simulink model "PE_weightstationary"  (R2022a)
settings: Solver=VariableStepAuto  StartTime=0.0  StopTime=20  RelTol=1e-3
values from neighbouring files (symbols this model uses):
  eta = 0.001    [array_2x2_input.m]
  num_layer = 4    [array_2x2_input.m]
undefined symbols (not defined in the file or in its folder): xc7k70tfbv676
libraries: hdlBasic x77, vmcUtilities x1
(part 1 of 2)
settings Model: Creator=gaozh  LastModifiedBy=gaozh

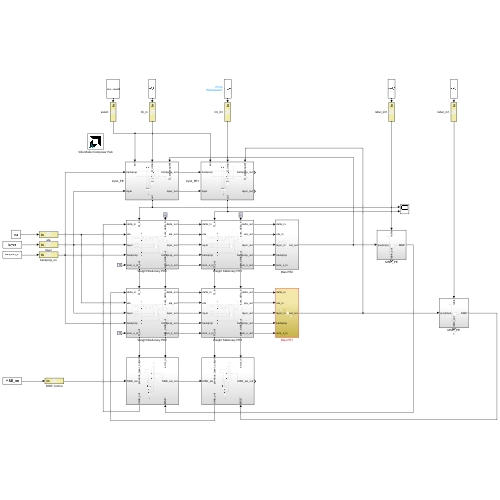
[thumbnail: Simulink's stored preview of the top-level diagram]
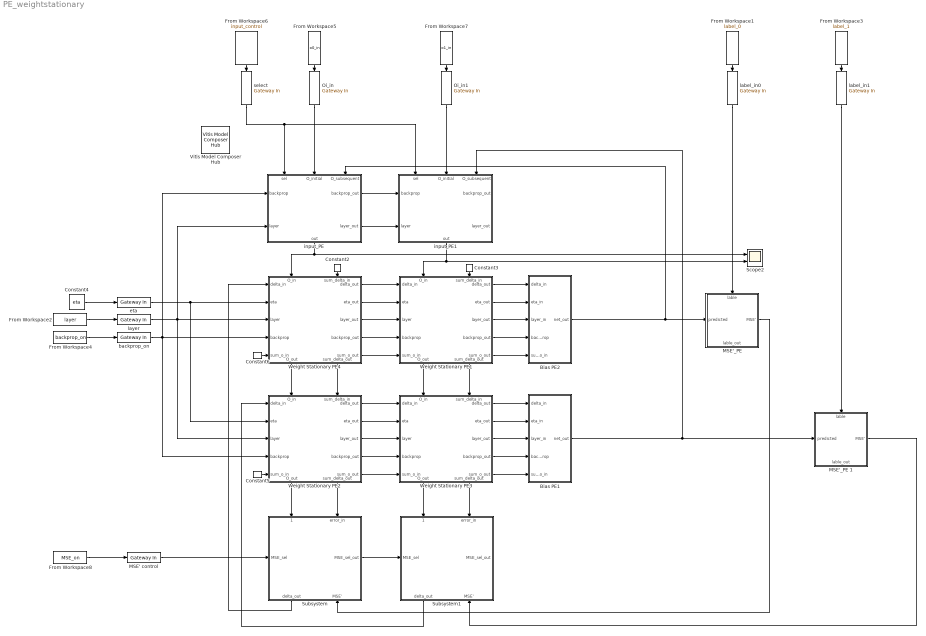
== system PE_weightstationary ==
  Bias PE1 : Subsystem
  Bias PE2 : Subsystem
  Constant{2..3,5..6} (4 alike) : hdlBasic/Constant  const=0  gui_display_data_type=Fixed-point  arith_type=Signed (2's comp)  n_bits=num_bits  bin_pt=frac_bits  preci_type=Single  exp_width=8  frac_width=24  explicit_period=off  period=1  XmcBlockStatus=1  maskContainerNames=tabcontainer1  block_type=constant  block_config=sysgen:Constant_config
  Constant4 : Constant  Value=eta
  From Workspace1 : FromWorkspace  VariableName=label_0
  From Workspace2 : FromWorkspace  VariableName=layer
  From Workspace3 : FromWorkspace  VariableName=label_1
  From Workspace4 : FromWorkspace  VariableName=backprop_on
  From Workspace5 : FromWorkspace  VariableName=o0_in
  From Workspace6 : FromWorkspace  VariableName=input_control
  From Workspace7 : FromWorkspace  VariableName=o1_in
  From Workspace8 : FromWorkspace  VariableName=MSE_on
  MSE' control : hdlBasic/Gateway In  gui_display_data_type=Boolean  arith_type=Boolean  n_bits=num_bits  bin_pt=0  preci_type=Single  exp_width=8  frac_width=24  rows=1  columns=1  quantization="Round  (unbiased: +/- Inf)"  overflow=Saturate  period=1  UseAsADC=off  ADCChannel='1'  interface=None  automatic_assignment=on  address_offset=hex2dec('00')  intf_name=''  intf_description=''  default_value=0  timing_constraint=None  locs_specified=off  LOCs={}  io_standard={}  inherit_from_input=off  hdl_port=on  XmcBlockStatus=1  maskContainerNames=group4  block_type=gatewayin  block_config=sysgen:gateway_in_config  block_width_w=590  block_height_w=620  block_width=640  block_height=850
  "MSE'_PE " : Subsystem
      settings: PortSchema="{\"entries\":[{\"content\":{\"sides\":[{\"content\":{\"connectorIds\":[\"In1\"]},\"type\":\"ConnectorPlacement.EquallySpacedRectSide\",\"uuid\":\"709b04f5-809b-41cc-9440-aba08c0e6347\"},{\"content\":{\"connectorIds\":[\"Out1\"],\"side\":\"RIGHT\"},\"type\":\"ConnectorPlacement.EquallySpacedRectSide\",\"uuid\":\"2a9bc808-cd74-4923-8833-c733d5b55101\"},{\"content\":{\"connectorIds\":[\"In2\"],\"side\":\"TOP\"},\"type\":\"ConnectorPlacement.EquallySpacedRectSide\",\"uuid\":\"1b9115af-72f6-4ff5-884d-2691fdb3b6f3\"},{\"content\":{\"connectorIds\":[\"Out2\"],\"side\":\"BOTTOM\"},\"type\":\"ConnectorPlacement.EquallySpacedRectSide\",\"uuid\":\"91ceb1b5-75ad-4997-b7e4-e67318ba19d7\"}]},\"type\":\"ConnectorPlacement.EquallySpacedConnector\",\"uuid\":\"1849f986-7f00-43c7-976b-1eef01c166bf\"}],\"packageUris\":[\"http://schema.mathworks.com/mf0/Connector/R2020b\"],\"version\":\"1.0\"}"
  MSE'_PE 1 : Subsystem
      settings: PortSchema="{\"entries\":[{\"content\":{\"sides\":[{\"content\":{\"connectorIds\":[\"In1\"]},\"type\":\"ConnectorPlacement.EquallySpacedRectSide\",\"uuid\":\"709b04f5-809b-41cc-9440-aba08c0e6347\"},{\"content\":{\"connectorIds\":[\"Out1\"],\"side\":\"RIGHT\"},\"type\":\"ConnectorPlacement.EquallySpacedRectSide\",\"uuid\":\"2a9bc808-cd74-4923-8833-c733d5b55101\"},{\"content\":{\"connectorIds\":[\"In2\"],\"side\":\"TOP\"},\"type\":\"ConnectorPlacement.EquallySpacedRectSide\",\"uuid\":\"1b9115af-72f6-4ff5-884d-2691fdb3b6f3\"},{\"content\":{\"connectorIds\":[\"Out2\"],\"side\":\"BOTTOM\"},\"type\":\"ConnectorPlacement.EquallySpacedRectSide\",\"uuid\":\"91ceb1b5-75ad-4997-b7e4-e67318ba19d7\"}]},\"type\":\"ConnectorPlacement.EquallySpacedConnector\",\"uuid\":\"1849f986-7f00-43c7-976b-1eef01c166bf\"}],\"packageUris\":[\"http://schema.mathworks.com/mf0/Connector/R2020b\"],\"version\":\"1.0\"}"
  Oi_in : hdlBasic/Gateway In  gui_display_data_type=Fixed-point  arith_type=Signed (2's comp)  n_bits=num_bits  bin_pt=frac_bits  preci_type=Single  exp_width=8  frac_width=24  rows=1  columns=1  quantization="Round  (unbiased: +/- Inf)"  overflow=Saturate  period=1  UseAsADC=off  ADCChannel='1'  interface=None  automatic_assignment=on  address_offset=hex2dec('00')  intf_name=''  intf_description=''  default_value=0  timing_constraint=None  locs_specified=off  LOCs={}  io_standard={}  inherit_from_input=off  hdl_port=on  XmcBlockStatus=1  maskContainerNames=group4  block_type=gatewayin  block_config=sysgen:gateway_in_config  block_width_w=590  block_height_w=620  block_width=640  block_height=850
  Oi_in1 : hdlBasic/Gateway In  gui_display_data_type=Fixed-point  arith_type=Signed (2's comp)  n_bits=num_bits  bin_pt=frac_bits  preci_type=Single  exp_width=8  frac_width=24  rows=1  columns=1  quantization="Round  (unbiased: +/- Inf)"  overflow=Saturate  period=1  UseAsADC=off  ADCChannel='1'  interface=None  automatic_assignment=on  address_offset=hex2dec('00')  intf_name=''  intf_description=''  default_value=0  timing_constraint=None  locs_specified=off  LOCs={}  io_standard={}  inherit_from_input=off  hdl_port=on  XmcBlockStatus=1  maskContainerNames=group4  block_type=gatewayin  block_config=sysgen:gateway_in_config  block_width_w=590  block_height_w=620  block_width=640  block_height=850
  Scope2 : Scope  NumInputPorts=2
  Subsystem : Subsystem
      settings: PortSchema="{\"entries\":[{\"content\":{\"sides\":[{\"content\":{\"connectorIds\":[\"In1\",\"In2\"]},\"type\":\"ConnectorPlacement.EquallySpacedRectSide\",\"uuid\":\"dbd75916-d643-4f7d-9fb6-d710889911bc\"},{\"content\":{\"connectorIds\":[\"Out1\",\"In4\"],\"side\":\"RIGHT\"},\"type\":\"ConnectorPlacement.EquallySpacedRectSide\",\"uuid\":\"bd082d37-a6ba-4642-a234-a4ee2405f373\"},{\"content\":{\"connectorIds\":[\"In3\"],\"side\":\"TOP\"},\"type\":\"ConnectorPlacement.EquallySpacedRectSide\",\"uuid\":\"2acf0bf3-92c2-4168-859e-2b2ecd63c261\"},{\"content\":{\"connectorIds\":[\"Out2\"],\"side\":\"BOTTOM\"},\"type\":\"ConnectorPlacement.EquallySpacedRectSide\",\"uuid\":\"570ce3db-e00a-4edd-9e75-c3405427573c\"}]},\"type\":\"ConnectorPlacement.EquallySpacedConnector\",\"uuid\":\"e2ba7bdc-2926-4fef-94e6-45d12da95ba7\"}],\"packageUris\":[\"http://schema.mathworks.com/mf0/Connector/R2020b\"],\"version\":\"1.0\"}"
  Subsystem1 : Subsystem
      settings: PortSchema="{\"entries\":[{\"content\":{\"sides\":[{\"content\":{\"connectorIds\":[\"In1\",\"In2\"]},\"type\":\"ConnectorPlacement.EquallySpacedRectSide\",\"uuid\":\"dbd75916-d643-4f7d-9fb6-d710889911bc\"},{\"content\":{\"connectorIds\":[\"Out1\",\"In4\"],\"side\":\"RIGHT\"},\"type\":\"ConnectorPlacement.EquallySpacedRectSide\",\"uuid\":\"bd082d37-a6ba-4642-a234-a4ee2405f373\"},{\"content\":{\"connectorIds\":[\"In3\"],\"side\":\"TOP\"},\"type\":\"ConnectorPlacement.EquallySpacedRectSide\",\"uuid\":\"2acf0bf3-92c2-4168-859e-2b2ecd63c261\"},{\"content\":{\"connectorIds\":[\"Out2\"],\"side\":\"BOTTOM\"},\"type\":\"ConnectorPlacement.EquallySpacedRectSide\",\"uuid\":\"570ce3db-e00a-4edd-9e75-c3405427573c\"}]},\"type\":\"ConnectorPlacement.EquallySpacedConnector\",\"uuid\":\"e2ba7bdc-2926-4fef-94e6-45d12da95ba7\"}],\"packageUris\":[\"http://schema.mathworks.com/mf0/Connector/R2020b\"],\"version\":\"1.0\"}"
  Vitis Model Composer Hub : vmcUtilities/Vitis Model Composer Hub  Tag=genX  CodeGeneration=off  TargetDirectory=./code  ExportType=AI Engines  IpVendor=xilinx.com  IpLibrary=hls  IpVersion=1.0  IpHWLanguage=Verilog  AieCompilerOptions={}  AieSimulatorOptions={}  CreateTestbench=off  TestbenchStackSize=10  RunAieSim=off  AieSimTimeout=50000  RunAieSimProfiling=off  LaunchVitisAnalyzer=off  PlotOutput=off  RunX86Sim=off  X86SimTimeout=10  GenHwImage=off  PlatformType=Not Specified  HwSystemType=Baremetal  HwValidationTarget=hw  ProjDevice=xc7k70tfbv676-1  ProjDevicePart=xc7k70tfbv676-1  SamplePeriod=-1  ClockFrequency=200  DataPathParallelism=1  xilinxfamily=kintex7  part=xc7k70t  speed=-1  package=fbv676  directory=./netlist  testbench=off  incr_netlist=off  synthesis_tool=Vivado  clock_wrapper=Clock Enables  dbl_ovrd=According to Block Masks  dcm_input_clock_period=10  sysclk_period=10  simulink_period=1  eval_field=0  IPInfoJsonString="{\"HDLSubsystem\":{\"SubsystemName\":\"PE_weightstationary\",\"IPName\":\"weight_pe\",\"IPLibrary\":\"VMC\",\"IPVendor\":\"User Company\",\"IPVersion\":\"1.0\"}}"  LogFileName=''  NThreads=4
  Weight Stationary PE1 : Subsystem
      settings: PortSchema="{\"entries\":[{\"content\":{\"sides\":[{\"content\":{\"connectorIds\":[\"In1\",\"In2\",\"In3\",\"In4\",\"In5\"]},\"type\":\"ConnectorPlacement.EquallySpacedRectSide\",\"uuid\":\"632a3ded-5b94-406e-b0d8-119737680536\"},{\"content\":{\"connectorIds\":[\"Out1\",\"Out2\",\"Out3\",\"Out4\",\"Out5\"],\"side\":\"RIGHT\"},\"type\":\"ConnectorPlacement.EquallySpacedRectSide\",\"uuid\":\"c449027c-81bc-4843-8994-fcad26195520\"},{\"content\":{\"connectorIds\":[\"In6\",\"In7\"],\"side\":\"TOP\"},\"type\":\"ConnectorPlacement.EquallySpacedRectSide\",\"uuid\":\"ce3d970d-7335-434e-bfbf-286e0c492397\"},{\"content\":{\"connectorIds\":[\"Out6\",\"Out7\"],\"side\":\"BOTTOM\"},\"type\":\"ConnectorPlacement.EquallySpacedRectSide\",\"uuid\":\"bc179919-f31d-4e0a-abc3-bb5ef913c3c8\"}]},\"type\":\"ConnectorPlacement.EquallySpacedConnector\",\"uuid\":\"cad1cfc6-1bed-4a03-a2df-30ebe0a8ed6f\"}],\"packageUris\":[\"http://schema.mathworks.com/mf0/Connector/R2020b\"],\"version\":\"1.0\"}"
  Weight Stationary PE2 : Subsystem
      settings: PortSchema="{\"entries\":[{\"content\":{\"sides\":[{\"content\":{\"connectorIds\":[\"In1\",\"In2\",\"In3\",\"In4\",\"In5\"]},\"type\":\"ConnectorPlacement.EquallySpacedRectSide\",\"uuid\":\"632a3ded-5b94-406e-b0d8-119737680536\"},{\"content\":{\"connectorIds\":[\"Out1\",\"Out2\",\"Out3\",\"Out4\",\"Out5\"],\"side\":\"RIGHT\"},\"type\":\"ConnectorPlacement.EquallySpacedRectSide\",\"uuid\":\"c449027c-81bc-4843-8994-fcad26195520\"},{\"content\":{\"connectorIds\":[\"In6\",\"In7\"],\"side\":\"TOP\"},\"type\":\"ConnectorPlacement.EquallySpacedRectSide\",\"uuid\":\"ce3d970d-7335-434e-bfbf-286e0c492397\"},{\"content\":{\"connectorIds\":[\"Out6\",\"Out7\"],\"side\":\"BOTTOM\"},\"type\":\"ConnectorPlacement.EquallySpacedRectSide\",\"uuid\":\"bc179919-f31d-4e0a-abc3-bb5ef913c3c8\"}]},\"type\":\"ConnectorPlacement.EquallySpacedConnector\",\"uuid\":\"cad1cfc6-1bed-4a03-a2df-30ebe0a8ed6f\"}],\"packageUris\":[\"http://schema.mathworks.com/mf0/Connector/R2020b\"],\"version\":\"1.0\"}"
  Weight Stationary PE3 : Subsystem
      settings: PortSchema="{\"entries\":[{\"content\":{\"sides\":[{\"content\":{\"connectorIds\":[\"In1\",\"In2\",\"In3\",\"In4\",\"In5\"]},\"type\":\"ConnectorPlacement.EquallySpacedRectSide\",\"uuid\":\"632a3ded-5b94-406e-b0d8-119737680536\"},{\"content\":{\"connectorIds\":[\"Out1\",\"Out2\",\"Out3\",\"Out4\",\"Out5\"],\"side\":\"RIGHT\"},\"type\":\"ConnectorPlacement.EquallySpacedRectSide\",\"uuid\":\"c449027c-81bc-4843-8994-fcad26195520\"},{\"content\":{\"connectorIds\":[\"In6\",\"In7\"],\"side\":\"TOP\"},\"type\":\"ConnectorPlacement.EquallySpacedRectSide\",\"uuid\":\"ce3d970d-7335-434e-bfbf-286e0c492397\"},{\"content\":{\"connectorIds\":[\"Out6\",\"Out7\"],\"side\":\"BOTTOM\"},\"type\":\"ConnectorPlacement.EquallySpacedRectSide\",\"uuid\":\"bc179919-f31d-4e0a-abc3-bb5ef913c3c8\"}]},\"type\":\"ConnectorPlacement.EquallySpacedConnector\",\"uuid\":\"cad1cfc6-1bed-4a03-a2df-30ebe0a8ed6f\"}],\"packageUris\":[\"http://schema.mathworks.com/mf0/Connector/R2020b\"],\"version\":\"1.0\"}"
  Weight Stationary PE4 : Subsystem
      settings: PortSchema="{\"entries\":[{\"content\":{\"sides\":[{\"content\":{\"connectorIds\":[\"In1\",\"In2\",\"In3\",\"In4\",\"In5\"]},\"type\":\"ConnectorPlacement.EquallySpacedRectSide\",\"uuid\":\"632a3ded-5b94-406e-b0d8-119737680536\"},{\"content\":{\"connectorIds\":[\"Out1\",\"Out2\",\"Out3\",\"Out4\",\"Out5\"],\"side\":\"RIGHT\"},\"type\":\"ConnectorPlacement.EquallySpacedRectSide\",\"uuid\":\"c449027c-81bc-4843-8994-fcad26195520\"},{\"content\":{\"connectorIds\":[\"In6\",\"In7\"],\"side\":\"TOP\"},\"type\":\"ConnectorPlacement.EquallySpacedRectSide\",\"uuid\":\"ce3d970d-7335-434e-bfbf-286e0c492397\"},{\"content\":{\"connectorIds\":[\"Out6\",\"Out7\"],\"side\":\"BOTTOM\"},\"type\":\"ConnectorPlacement.EquallySpacedRectSide\",\"uuid\":\"bc179919-f31d-4e0a-abc3-bb5ef913c3c8\"}]},\"type\":\"ConnectorPlacement.EquallySpacedConnector\",\"uuid\":\"cad1cfc6-1bed-4a03-a2df-30ebe0a8ed6f\"}],\"packageUris\":[\"http://schema.mathworks.com/mf0/Connector/R2020b\"],\"version\":\"1.0\"}"
  backprop_on : hdlBasic/Gateway In  gui_display_data_type=Boolean  arith_type=Boolean  n_bits=num_bits  bin_pt=0  preci_type=Single  exp_width=8  frac_width=24  rows=1  columns=1  quantization="Round  (unbiased: +/- Inf)"  overflow=Saturate  period=1  UseAsADC=off  ADCChannel='1'  interface=None  automatic_assignment=on  address_offset=hex2dec('00')  intf_name=''  intf_description=''  default_value=0  timing_constraint=None  locs_specified=off  LOCs={}  io_standard={}  inherit_from_input=off  hdl_port=on  XmcBlockStatus=1  maskContainerNames=group4  block_type=gatewayin  block_config=sysgen:gateway_in_config  block_width_w=590  block_height_w=620  block_width=640  block_height=850
  eta : hdlBasic/Gateway In  gui_display_data_type=Fixed-point  arith_type=Signed (2's comp)  n_bits=num_bits  bin_pt=frac_bits  preci_type=Single  exp_width=8  frac_width=24  rows=1  columns=1  quantization="Round  (unbiased: +/- Inf)"  overflow=Saturate  period=1  UseAsADC=off  ADCChannel='1'  interface=None  automatic_assignment=on  address_offset=hex2dec('00')  intf_name=''  intf_description=''  default_value=0  timing_constraint=None  locs_specified=off  LOCs={}  io_standard={}  inherit_from_input=off  hdl_port=on  XmcBlockStatus=1  maskContainerNames=group4  block_type=gatewayin  block_config=sysgen:gateway_in_config  block_width_w=590  block_height_w=620  block_width=640  block_height=850
  input_PE : Subsystem
      settings: PortSchema="{\"entries\":[{\"content\":{\"sides\":[{\"content\":{\"connectorIds\":[\"In1\",\"In2\",\"In3\"]},\"type\":\"ConnectorPlacement.EquallySpacedRectSide\",\"uuid\":\"a4b85e5c-8615-4c6f-a824-e1b9d50a6a2f\"},{\"content\":{\"connectorIds\":[\"Out1\"],\"side\":\"RIGHT\"},\"type\":\"ConnectorPlacement.EquallySpacedRectSide\",\"uuid\":\"8e5fd073-8d4c-453d-b945-af756751d2bd\"},{\"content\":{\"connectorIds\":[\"In4\",\"In5\"],\"side\":\"TOP\"},\"type\":\"ConnectorPlacement.EquallySpacedRectSide\",\"uuid\":\"5eacf5cb-78e1-4bbb-935c-2d6844e409c1\"},{\"content\":{\"connectorIds\":[\"Out2\",\"Out3\"],\"side\":\"BOTTOM\"},\"type\":\"ConnectorPlacement.EquallySpacedRectSide\",\"uuid\":\"56810a3a-92d6-45f4-9b79-95487ce57caf\"}]},\"type\":\"ConnectorPlacement.EquallySpacedConnector\",\"uuid\":\"b8112838-ef89-45c9-af16-03e0b6ed3724\"}],\"packageUris\":[\"http://schema.mathworks.com/mf0/Connector/R2020b\"],\"version\":\"1.0\"}"
  input_PE1 : Subsystem
      settings: PortSchema="{\"entries\":[{\"content\":{\"sides\":[{\"content\":{\"connectorIds\":[\"In1\",\"In2\",\"In3\"]},\"type\":\"ConnectorPlacement.EquallySpacedRectSide\",\"uuid\":\"a4b85e5c-8615-4c6f-a824-e1b9d50a6a2f\"},{\"content\":{\"connectorIds\":[\"Out1\"],\"side\":\"RIGHT\"},\"type\":\"ConnectorPlacement.EquallySpacedRectSide\",\"uuid\":\"8e5fd073-8d4c-453d-b945-af756751d2bd\"},{\"content\":{\"connectorIds\":[\"In4\",\"In5\"],\"side\":\"TOP\"},\"type\":\"ConnectorPlacement.EquallySpacedRectSide\",\"uuid\":\"5eacf5cb-78e1-4bbb-935c-2d6844e409c1\"},{\"content\":{\"connectorIds\":[\"Out2\",\"Out3\"],\"side\":\"BOTTOM\"},\"type\":\"ConnectorPlacement.EquallySpacedRectSide\",\"uuid\":\"56810a3a-92d6-45f4-9b79-95487ce57caf\"}]},\"type\":\"ConnectorPlacement.EquallySpacedConnector\",\"uuid\":\"b8112838-ef89-45c9-af16-03e0b6ed3724\"}],\"packageUris\":[\"http://schema.mathworks.com/mf0/Connector/R2020b\"],\"version\":\"1.0\"}"
  label_in0 : hdlBasic/Gateway In  gui_display_data_type=Fixed-point  arith_type=Signed (2's comp)  n_bits=num_bits  bin_pt=frac_bits  preci_type=Single  exp_width=8  frac_width=24  rows=1  columns=1  quantization="Round  (unbiased: +/- Inf)"  overflow=Saturate  period=1  UseAsADC=off  ADCChannel='1'  interface=None  automatic_assignment=on  address_offset=hex2dec('00')  intf_name=''  intf_description=''  default_value=0  timing_constraint=None  locs_specified=off  LOCs={}  io_standard={}  inherit_from_input=off  hdl_port=on  XmcBlockStatus=1  maskContainerNames=group4  block_type=gatewayin  block_config=sysgen:gateway_in_config  block_width_w=590  block_height_w=620  block_width=640  block_height=850
  label_in1 : hdlBasic/Gateway In  gui_display_data_type=Fixed-point  arith_type=Signed (2's comp)  n_bits=num_bits  bin_pt=frac_bits  preci_type=Single  exp_width=8  frac_width=24  rows=1  columns=1  quantization="Round  (unbiased: +/- Inf)"  overflow=Saturate  period=1  UseAsADC=off  ADCChannel='1'  interface=None  automatic_assignment=on  address_offset=hex2dec('00')  intf_name=''  intf_description=''  default_value=0  timing_constraint=None  locs_specified=off  LOCs={}  io_standard={}  inherit_from_input=off  hdl_port=on  XmcBlockStatus=1  maskContainerNames=group4  block_type=gatewayin  block_config=sysgen:gateway_in_config  block_width_w=590  block_height_w=620  block_width=640  block_height=850
  layer : hdlBasic/Gateway In  gui_display_data_type=Fixed-point  arith_type=Unsigned  n_bits=ceil(log2(num_layer))  bin_pt=0  preci_type=Single  exp_width=8  frac_width=24  rows=1  columns=1  quantization="Round  (unbiased: +/- Inf)"  overflow=Saturate  period=1  UseAsADC=off  ADCChannel='1'  interface=None  automatic_assignment=on  address_offset=hex2dec('00')  intf_name=''  intf_description=''  default_value=0  timing_constraint=None  locs_specified=off  LOCs={}  io_standard={}  inherit_from_input=off  hdl_port=on  XmcBlockStatus=1  maskContainerNames=group4  block_type=gatewayin  block_config=sysgen:gateway_in_config  block_width_w=590  block_height_w=620  block_width=640  block_height=850
  select : hdlBasic/Gateway In  gui_display_data_type=Fixed-point  arith_type=Unsigned  n_bits=2  bin_pt=0  preci_type=Single  exp_width=8  frac_width=24  rows=1  columns=1  quantization="Round  (unbiased: +/- Inf)"  overflow=Flag as error  period=1  UseAsADC=off  ADCChannel='1'  interface=None  automatic_assignment=on  address_offset=hex2dec('00')  intf_name=''  intf_description=''  default_value=0  timing_constraint=None  locs_specified=off  LOCs={}  io_standard={}  inherit_from_input=off  hdl_port=on  XmcBlockStatus=1  maskContainerNames=group4  block_type=gatewayin  block_config=sysgen:gateway_in_config  block_width_w=590  block_height_w=620  block_width=640  block_height=850
  wires:
  Constant4/1 -> eta/1
  From Workspace4/1 -> backprop_on/1
  From Workspace5/1 -> Oi_in/1
  Weight Stationary PE4/1(delta_out) -> Weight Stationary PE1/1(delta_in)
  Weight Stationary PE4/2(eta_out) -> Weight Stationary PE1/2(eta)
  Weight Stationary PE4/3(layer_out) -> Weight Stationary PE1/3(layer)
  Weight Stationary PE4/5(sum_o_out) -> Weight Stationary PE1/5(sum_o_in)
  Weight Stationary PE4/4(backprop_out) -> Weight Stationary PE1/4(backprop)
  Weight Stationary PE1/6(O_out) -> Weight Stationary PE3/6(O_in)
  Weight Stationary PE4/6(O_out) -> Weight Stationary PE2/6(O_in)
  Weight Stationary PE4/7(sum_delta_out) -> Weight Stationary PE2/7(sum_delta_in)
  Weight Stationary PE2/1(delta_out) -> Weight Stationary PE3/1(delta_in)
  Weight Stationary PE2/2(eta_out) -> Weight Stationary PE3/2(eta)
  Weight Stationary PE2/3(layer_out) -> Weight Stationary PE3/3(layer)
  Weight Stationary PE2/4(backprop_out) -> Weight Stationary PE3/4(backprop)
  Weight Stationary PE2/5(sum_o_out) -> Weight Stationary PE3/5(sum_o_in)
  eta/1 -> Weight Stationary PE2/2(eta), Weight Stationary PE4/2(eta)
  backprop_on/1 -> input_PE/4(backprop), Weight Stationary PE2/4(backprop), Weight Stationary PE4/4(backprop)
  layer/1 -> Weight Stationary PE2/3(layer), input_PE/5(layer), Weight Stationary PE4/3(layer)
  From Workspace7/1 -> Oi_in1/1
  From Workspace2/1 -> layer/1
  Weight Stationary PE1/7(sum_delta_out) -> Weight Stationary PE3/7(sum_delta_in)
  input_PE1/1(out) -> Weight Stationary PE1/6(O_in), Scope2/2
  From Workspace6/1 -> select/1
  select/1 -> input_PE1/1(sel), input_PE/1(sel)
  Weight Stationary PE1/1(delta_out) -> Bias PE2/1(delta_in)
  Weight Stationary PE1/2(eta_out) -> Bias PE2/2(eta_in)
  Weight Stationary PE1/3(layer_out) -> Bias PE2/3(layer_in)
  Weight Stationary PE1/4(backprop_out) -> Bias PE2/4(backprop)
  Weight Stationary PE1/5(sum_o_out) -> Bias PE2/5(sum_o_in)
  Weight Stationary PE3/1(delta_out) -> Bias PE1/1(delta_in)
  Weight Stationary PE3/2(eta_out) -> Bias PE1/2(eta_in)
  Weight Stationary PE3/3(layer_out) -> Bias PE1/3(layer_in)
  Weight Stationary PE3/4(backprop_out) -> Bias PE1/4(backprop)
  Weight Stationary PE3/5(sum_o_out) -> Bias PE1/5(sum_o_in)
  Constant2/1 -> Weight Stationary PE4/7(sum_delta_in)
  Constant3/1 -> Weight Stationary PE1/7(sum_delta_in)
  Constant5/1 -> Weight Stationary PE2/5(sum_o_in)
  Constant6/1 -> Weight Stationary PE4/5(sum_o_in)
  Bias PE1/1(net_out) -> MSE'_PE 1/1(predicted), input_PE1/3(O_subsequent)
  input_PE/1(out) -> Weight Stationary PE4/6(O_in), Scope2/1
  Oi_in/1 -> input_PE/2(O_initial)
  Bias PE2/1(net_out) -> input_PE/3(O_subsequent), "MSE'_PE "/1(predicted)
  input_PE/3(layer_out) -> input_PE1/5(layer)
  input_PE/2(backprop_out) -> input_PE1/4(backprop)
  Oi_in1/1 -> input_PE1/2(O_initial)
  label_in0/1 -> "MSE'_PE "/2(lable)
  From Workspace1/1 -> label_in0/1
  MSE'_PE 1/1(MSE') -> Subsystem1/4(MSE')
  From Workspace8/1 -> MSE' control/1
  "MSE'_PE "/1(MSE') -> Subsystem/4(MSE')
  Weight Stationary PE2/6(O_out) -> Subsystem/1(previous_layer_output)
  Weight Stationary PE2/7(sum_delta_out) -> Subsystem/2(error_in)
  MSE' control/1 -> Subsystem/3(MSE_sel)
  Subsystem/1(delta_out) -> Weight Stationary PE4/1(delta_in)
  Weight Stationary PE3/6(O_out) -> Subsystem1/1(previous_layer_output)
  Weight Stationary PE3/7(sum_delta_out) -> Subsystem1/2(error_in)
  Subsystem/2(MSE_sel_out) -> Subsystem1/3(MSE_sel)
  Subsystem1/1(delta_out) -> Weight Stationary PE2/1(delta_in)
  label_in1/1 -> MSE'_PE 1/2(lable)
  From Workspace3/1 -> label_in1/1

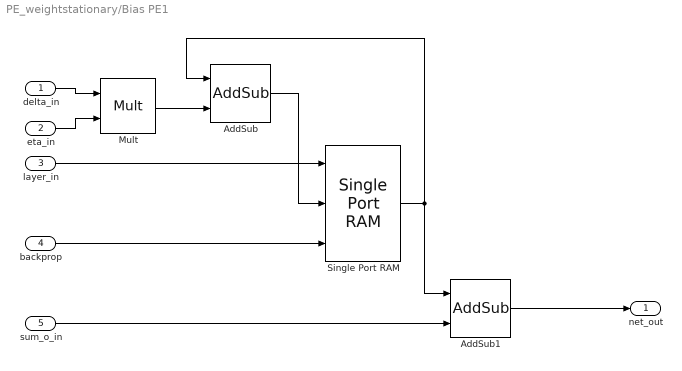
== system PE_weightstationary/Bias PE1 ==
  delta_in : Inport
  eta_in : Inport  Port=2
  layer_in : Inport  Port=3
  backprop : Inport  Port=4
  sum_o_in : Inport  Port=5
  AddSub : hdlBasic/AddSub  mode=Subtraction  use_carryin=off  use_carryout=off  en=off  latency=0  precision=User Defined  arith_type="Signed  (2's comp)"  n_bits=num_bits  bin_pt=frac_bits  quantization=Truncate  overflow=Saturate  use_behavioral_HDL=off  hw_selection=Fabric  pipelined=off  XmcBlockStatus=1  maskContainerNames=tabcontainer1  block_type=addsub  block_config=sysgen:Addsub_config
  AddSub1 : hdlBasic/AddSub  mode=Addition  use_carryin=off  use_carryout=off  en=off  latency=0  precision=User Defined  arith_type="Signed  (2's comp)"  n_bits=num_bits  bin_pt=frac_bits  quantization=Truncate  overflow=Saturate  use_behavioral_HDL=off  hw_selection=Fabric  pipelined=off  XmcBlockStatus=1  maskContainerNames=tabcontainer1  block_type=addsub  block_config=sysgen:Addsub_config
  Mult : hdlBasic/Mult  precision=User Defined  arith_type="Signed  (2's comp)"  n_bits=num_bits  bin_pt=frac_bits  quantization=Truncate  overflow=Saturate  en=off  latency=0  use_behavioral_HDL=off  opt=Speed  use_embedded=on  optimum_pipeline=off  pipeline=on  use_rpm=on  placement_style=Triangular  XmcBlockStatus=1  maskContainerNames=group1  block_type=mult  block_config=sysgen:Mult_config  block_width=598  block_height=876
  Single Port RAM : hdlBasic/Single Port RAM  depth=num_layer  initVector=initial_bias  distributed_mem=Block RAM  write_mode=Read After Write  rst=off  init_reg=0  en=off  optimize_latency=off  latency=1  optimize=Area  dbl_ovrd=off  simulation_type=fast_sim  XmcBlockStatus=1  maskContainerNames=tabcontainer1  block_type=spram  block_config=sysgen:SPRAM_config
  net_out : Outport
  wires:
  layer_in/1 -> Single Port RAM/1
  delta_in/1 -> Mult/1
  Single Port RAM/1 -> AddSub1/1, AddSub/1
  eta_in/1 -> Mult/2
  backprop/1 -> Single Port RAM/3
  sum_o_in/1 -> AddSub1/2
  Mult/1 -> AddSub/2
  AddSub/1 -> Single Port RAM/2
  AddSub1/1 -> net_out/1

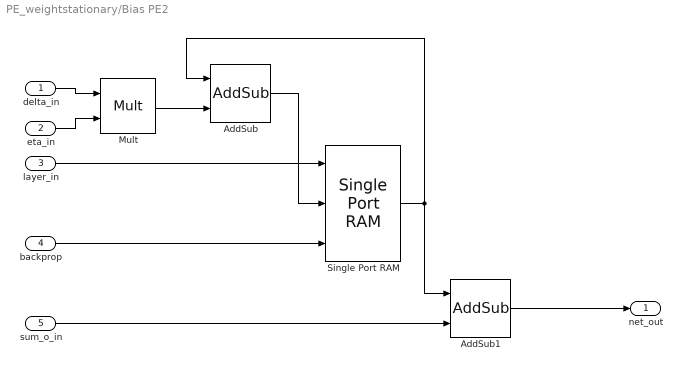
== system PE_weightstationary/Bias PE2 ==
  delta_in : Inport
  eta_in : Inport  Port=2
  layer_in : Inport  Port=3
  backprop : Inport  Port=4
  sum_o_in : Inport  Port=5
  AddSub : hdlBasic/AddSub  mode=Subtraction  use_carryin=off  use_carryout=off  en=off  latency=0  precision=User Defined  arith_type="Signed  (2's comp)"  n_bits=num_bits  bin_pt=frac_bits  quantization=Truncate  overflow=Saturate  use_behavioral_HDL=off  hw_selection=Fabric  pipelined=off  XmcBlockStatus=1  maskContainerNames=tabcontainer1  block_type=addsub  block_config=sysgen:Addsub_config
  AddSub1 : hdlBasic/AddSub  mode=Addition  use_carryin=off  use_carryout=off  en=off  latency=0  precision=User Defined  arith_type="Signed  (2's comp)"  n_bits=num_bits  bin_pt=frac_bits  quantization=Truncate  overflow=Saturate  use_behavioral_HDL=off  hw_selection=Fabric  pipelined=off  XmcBlockStatus=1  maskContainerNames=tabcontainer1  block_type=addsub  block_config=sysgen:Addsub_config
  Mult : hdlBasic/Mult  precision=User Defined  arith_type="Signed  (2's comp)"  n_bits=num_bits  bin_pt=frac_bits  quantization=Truncate  overflow=Saturate  en=off  latency=0  use_behavioral_HDL=off  opt=Speed  use_embedded=on  optimum_pipeline=off  pipeline=on  use_rpm=on  placement_style=Triangular  XmcBlockStatus=1  maskContainerNames=group1  block_type=mult  block_config=sysgen:Mult_config  block_width=598  block_height=876
  Single Port RAM : hdlBasic/Single Port RAM  depth=num_layer  initVector=initial_bias  distributed_mem=Block RAM  write_mode=Read After Write  rst=off  init_reg=0  en=off  optimize_latency=off  latency=1  optimize=Area  dbl_ovrd=off  simulation_type=fast_sim  XmcBlockStatus=1  maskContainerNames=tabcontainer1  block_type=spram  block_config=sysgen:SPRAM_config
  net_out : Outport
  wires:
  layer_in/1 -> Single Port RAM/1
  delta_in/1 -> Mult/1
  Single Port RAM/1 -> AddSub1/1, AddSub/1
  eta_in/1 -> Mult/2
  backprop/1 -> Single Port RAM/3
  sum_o_in/1 -> AddSub1/2
  Mult/1 -> AddSub/2
  AddSub/1 -> Single Port RAM/2
  AddSub1/1 -> net_out/1

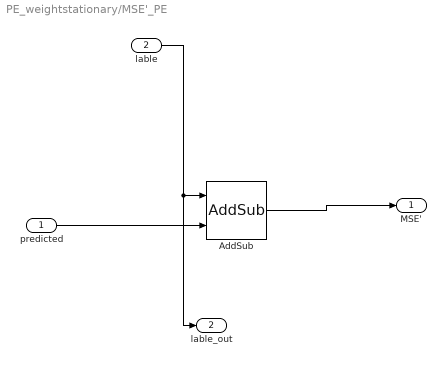
== system PE_weightstationary/MSE'_PE  ==
  predicted : Inport
  lable : Inport  Port=2
  AddSub : hdlBasic/AddSub  mode=Subtraction  use_carryin=off  use_carryout=off  en=off  latency=0  precision=Full  arith_type=Unsigned  n_bits=16  bin_pt=14  quantization=Truncate  overflow=Wrap  use_behavioral_HDL=off  hw_selection=Fabric  pipelined=off  XmcBlockStatus=1  maskContainerNames=tabcontainer1  block_type=addsub  block_config=sysgen:Addsub_config
  MSE' : Outport
  lable_out : Outport  Port=2
  wires:
  lable/1 -> lable_out/1, AddSub/1
  AddSub/1 -> MSE'/1
  predicted/1 -> AddSub/2

== system PE_weightstationary/MSE'_PE 1 ==
  predicted : Inport
  lable : Inport  Port=2
  AddSub : hdlBasic/AddSub  mode=Subtraction  use_carryin=off  use_carryout=off  en=off  latency=0  precision=Full  arith_type=Unsigned  n_bits=16  bin_pt=14  quantization=Truncate  overflow=Wrap  use_behavioral_HDL=off  hw_selection=Fabric  pipelined=off  XmcBlockStatus=1  maskContainerNames=tabcontainer1  block_type=addsub  block_config=sysgen:Addsub_config
  MSE' : Outport
  lable_out : Outport  Port=2
  wires:
  lable/1 -> lable_out/1, AddSub/1
  AddSub/1 -> MSE'/1
  predicted/1 -> AddSub/2

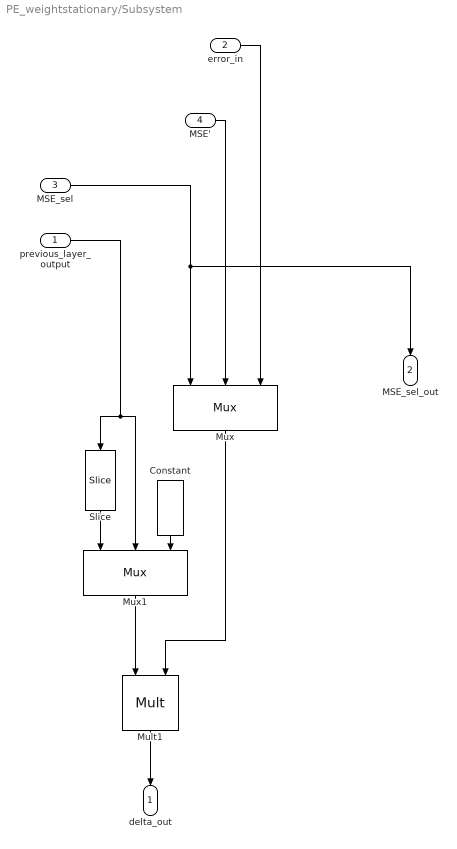
== system PE_weightstationary/Subsystem ==
  previous_layer_output : Inport
  error_in : Inport  Port=2
  MSE_sel : Inport  Port=3
  MSE' : Inport  Port=4
  Constant : hdlBasic/Constant  const=0  gui_display_data_type=Fixed-point  arith_type=Signed (2's comp)  n_bits=num_bits  bin_pt=frac_bits  preci_type=Single  exp_width=8  frac_width=24  explicit_period=off  period=1  XmcBlockStatus=1  maskContainerNames=tabcontainer1  block_type=constant  block_config=sysgen:Constant_config
  Mult1 : hdlBasic/Mult  precision=User Defined  arith_type="Signed  (2's comp)"  n_bits=num_bits  bin_pt=3  quantization=Truncate  overflow=Wrap  en=off  latency=0  use_behavioral_HDL=off  opt=Speed  use_embedded=on  optimum_pipeline=off  pipeline=on  use_rpm=on  placement_style=Triangular  XmcBlockStatus=1  maskContainerNames=group1  block_type=mult  block_config=sysgen:Mult_config  block_width=598  block_height=876
  Mux : hdlBasic/Mux  inputs=2  en=off  latency=1  precision=User Defined  arith_type="Signed  (2's comp)"  n_bits=num_bits  bin_pt=frac_bits  quantization=Truncate  overflow=Saturate  XmcBlockStatus=1  maskContainerNames=tabcontainer1  block_type=mux  block_config=sysgen:Mux_config
  Mux1 : hdlBasic/Mux  inputs=2  en=off  latency=1  precision=User Defined  arith_type="Signed  (2's comp)"  n_bits=num_bits  bin_pt=frac_bits  quantization=Truncate  overflow=Saturate  XmcBlockStatus=1  maskContainerNames=tabcontainer1  block_type=mux  block_config=sysgen:Mux_config
  Slice : hdlBasic/Slice  nbits=1  boolean_output=on  mode=Upper Bit Location + Width  bit1=0  base1=MSB of Input  bit0=0  base0=LSB of Input  XmcBlockStatus=1  maskContainerNames=group1  block_type=slice  block_config=sysgen:Slice_config
  delta_out : Outport
  MSE_sel_out : Outport  Port=2
  wires:
  Constant/1 -> Mux1/3
  Mux1/1 -> Mult1/1
  previous_layer_output/1 -> Slice/1, Mux1/2
  Mult1/1 -> delta_out/1
  error_in/1 -> Mux/3
  MSE'/1 -> Mux/2
  Mux/1 -> Mult1/2
  Slice/1 -> Mux1/1
  MSE_sel/1 -> MSE_sel_out/1, Mux/1

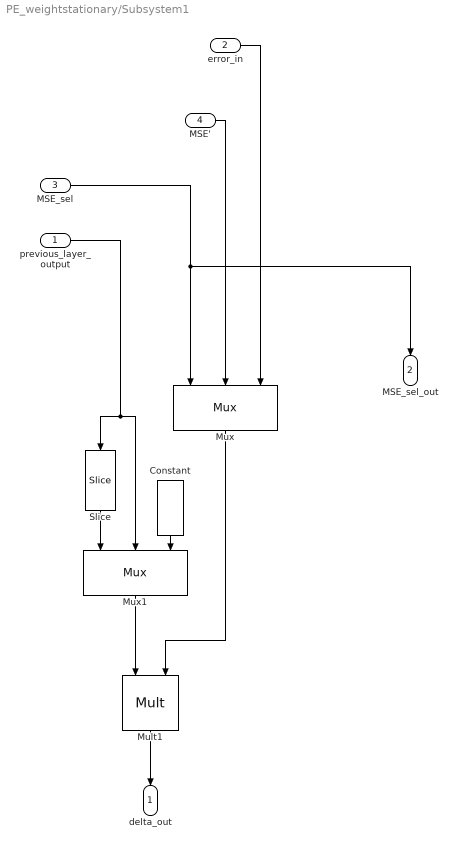
== system PE_weightstationary/Subsystem1 ==
  previous_layer_output : Inport
  error_in : Inport  Port=2
  MSE_sel : Inport  Port=3
  MSE' : Inport  Port=4
  Constant : hdlBasic/Constant  const=0  gui_display_data_type=Fixed-point  arith_type=Signed (2's comp)  n_bits=num_bits  bin_pt=frac_bits  preci_type=Single  exp_width=8  frac_width=24  explicit_period=off  period=1  XmcBlockStatus=1  maskContainerNames=tabcontainer1  block_type=constant  block_config=sysgen:Constant_config
  Mult1 : hdlBasic/Mult  precision=User Defined  arith_type="Signed  (2's comp)"  n_bits=num_bits  bin_pt=3  quantization=Truncate  overflow=Wrap  en=off  latency=0  use_behavioral_HDL=off  opt=Speed  use_embedded=on  optimum_pipeline=off  pipeline=on  use_rpm=on  placement_style=Triangular  XmcBlockStatus=1  maskContainerNames=group1  block_type=mult  block_config=sysgen:Mult_config  block_width=598  block_height=876
  Mux : hdlBasic/Mux  inputs=2  en=off  latency=1  precision=User Defined  arith_type="Signed  (2's comp)"  n_bits=num_bits  bin_pt=frac_bits  quantization=Truncate  overflow=Saturate  XmcBlockStatus=1  maskContainerNames=tabcontainer1  block_type=mux  block_config=sysgen:Mux_config
  Mux1 : hdlBasic/Mux  inputs=2  en=off  latency=1  precision=User Defined  arith_type="Signed  (2's comp)"  n_bits=num_bits  bin_pt=frac_bits  quantization=Truncate  overflow=Saturate  XmcBlockStatus=1  maskContainerNames=tabcontainer1  block_type=mux  block_config=sysgen:Mux_config
  Slice : hdlBasic/Slice  nbits=1  boolean_output=on  mode=Upper Bit Location + Width  bit1=0  base1=MSB of Input  bit0=0  base0=LSB of Input  XmcBlockStatus=1  maskContainerNames=group1  block_type=slice  block_config=sysgen:Slice_config
  delta_out : Outport
  MSE_sel_out : Outport  Port=2
  wires:
  Constant/1 -> Mux1/3
  Mux1/1 -> Mult1/1
  previous_layer_output/1 -> Slice/1, Mux1/2
  Mult1/1 -> delta_out/1
  error_in/1 -> Mux/3
  MSE'/1 -> Mux/2
  Mux/1 -> Mult1/2
  Slice/1 -> Mux1/1
  MSE_sel/1 -> MSE_sel_out/1, Mux/1

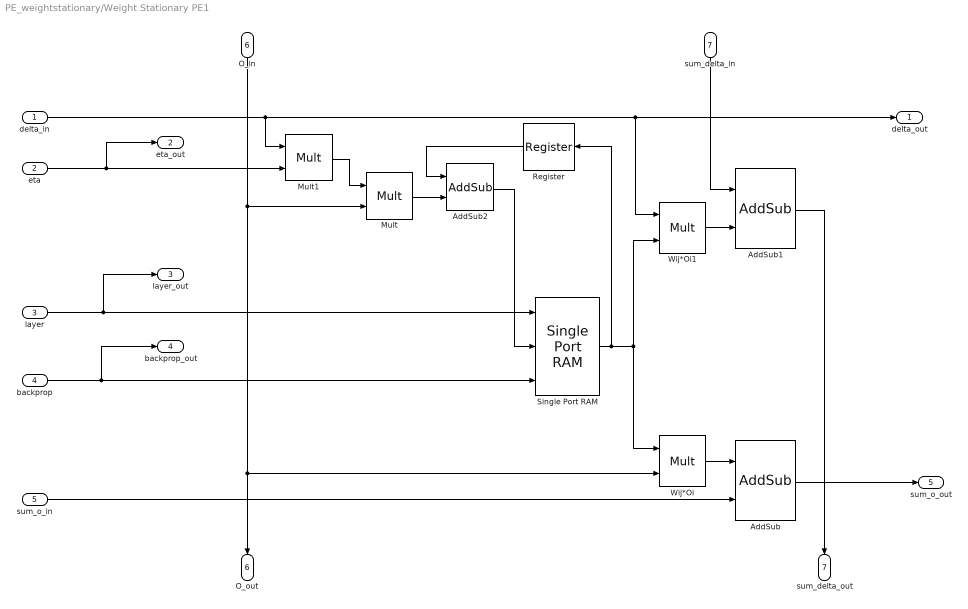
== system PE_weightstationary/Weight Stationary PE1 ==
  delta_in : Inport
  eta : Inport  Port=2
  layer : Inport  Port=3
  backprop : Inport  Port=4
  sum_o_in : Inport  Port=5
  O_in : Inport  Port=6
  sum_delta_in : Inport  Port=7
  AddSub : hdlBasic/AddSub  mode=Addition  use_carryin=off  use_carryout=off  en=off  latency=0  precision=User Defined  arith_type="Signed  (2's comp)"  n_bits=num_bits  bin_pt=frac_bits  quantization=Truncate  overflow=Saturate  use_behavioral_HDL=off  hw_selection=Fabric  pipelined=off  XmcBlockStatus=1  maskContainerNames=tabcontainer1  block_type=addsub  block_config=sysgen:Addsub_config
  AddSub1 : hdlBasic/AddSub  mode=Addition  use_carryin=off  use_carryout=off  en=off  latency=0  precision=User Defined  arith_type="Signed  (2's comp)"  n_bits=num_bits  bin_pt=frac_bits  quantization=Truncate  overflow=Saturate  use_behavioral_HDL=off  hw_selection=Fabric  pipelined=off  XmcBlockStatus=1  maskContainerNames=tabcontainer1  block_type=addsub  block_config=sysgen:Addsub_config
  AddSub2 : hdlBasic/AddSub  mode=Subtraction  use_carryin=off  use_carryout=off  en=off  latency=0  precision=User Defined  arith_type="Signed  (2's comp)"  n_bits=num_bits  bin_pt=frac_bits  quantization=Truncate  overflow=Wrap  use_behavioral_HDL=off  hw_selection=Fabric  pipelined=off  XmcBlockStatus=1  maskContainerNames=tabcontainer1  block_type=addsub  block_config=sysgen:Addsub_config
  Mult : hdlBasic/Mult  precision=User Defined  arith_type="Signed  (2's comp)"  n_bits=num_bits  bin_pt=frac_bits  quantization=Truncate  overflow=Saturate  en=off  latency=0  use_behavioral_HDL=off  opt=Speed  use_embedded=on  optimum_pipeline=off  pipeline=on  use_rpm=on  placement_style=Triangular  XmcBlockStatus=1  maskContainerNames=group1  block_type=mult  block_config=sysgen:Mult_config  block_width=598  block_height=876
  Mult1 : hdlBasic/Mult  precision=User Defined  arith_type="Signed  (2's comp)"  n_bits=num_bits  bin_pt=frac_bits  quantization=Truncate  overflow=Saturate  en=off  latency=0  use_behavioral_HDL=off  opt=Speed  use_embedded=on  optimum_pipeline=off  pipeline=on  use_rpm=on  placement_style=Triangular  XmcBlockStatus=1  maskContainerNames=group1  block_type=mult  block_config=sysgen:Mult_config  block_width=598  block_height=876
  Register : hdlBasic/Register  init=0  rst=off  en=off  XmcBlockStatus=1  maskContainerNames=tabcontainer1  block_type=register  block_config=sysgen:Register_config
  Single Port RAM : hdlBasic/Single Port RAM  depth=num_layer  initVector=initial_weight  distributed_mem=Block RAM  write_mode=Read After Write  rst=off  init_reg=0  en=off  optimize_latency=off  latency=1  optimize=Area  dbl_ovrd=off  simulation_type=fast_sim  XmcBlockStatus=1  maskContainerNames=tabcontainer1  block_type=spram  block_config=sysgen:SPRAM_config
  Wij*Oi : hdlBasic/Mult  precision=User Defined  arith_type="Signed  (2's comp)"  n_bits=num_bits  bin_pt=frac_bits  quantization=Truncate  overflow=Saturate  en=off  latency=0  use_behavioral_HDL=off  opt=Speed  use_embedded=on  optimum_pipeline=off  pipeline=on  use_rpm=on  placement_style=Triangular  XmcBlockStatus=1  maskContainerNames=group1  block_type=mult  block_config=sysgen:Mult_config  block_width=598  block_height=876
  Wij*Oi1 : hdlBasic/Mult  precision=User Defined  arith_type="Signed  (2's comp)"  n_bits=num_bits  bin_pt=frac_bits  quantization=Truncate  overflow=Saturate  en=off  latency=0  use_behavioral_HDL=off  opt=Speed  use_embedded=on  optimum_pipeline=off  pipeline=on  use_rpm=on  placement_style=Triangular  XmcBlockStatus=1  maskContainerNames=group1  block_type=mult  block_config=sysgen:Mult_config  block_width=598  block_height=876
  delta_out : Outport
  eta_out : Outport  Port=2
  layer_out : Outport  Port=3
  backprop_out : Outport  Port=4
  sum_o_out : Outport  Port=5
  O_out : Outport  Port=6
  sum_delta_out : Outport  Port=7
  wires:
  Wij*Oi1/1 -> AddSub1/2
  O_in/1 -> Wij*Oi/2, O_out/1, Mult/2
  Single Port RAM/1 -> Wij*Oi1/2, Wij*Oi/1, Register/1
  Wij*Oi/1 -> AddSub/1
  Mult/1 -> AddSub2/2
  AddSub1/1 -> sum_delta_out/1
  AddSub2/1 -> Single Port RAM/2
  Mult1/1 -> Mult/1
  delta_in/1 -> delta_out/1, Wij*Oi1/1, Mult1/1
  sum_o_in/1 -> AddSub/2
  AddSub/1 -> sum_o_out/1
  eta/1 -> Mult1/2, eta_out/1
  sum_delta_in/1 -> AddSub1/1
  backprop/1 -> Single Port RAM/3, backprop_out/1
  Register/1 -> AddSub2/1
  layer/1 -> Single Port RAM/1, layer_out/1

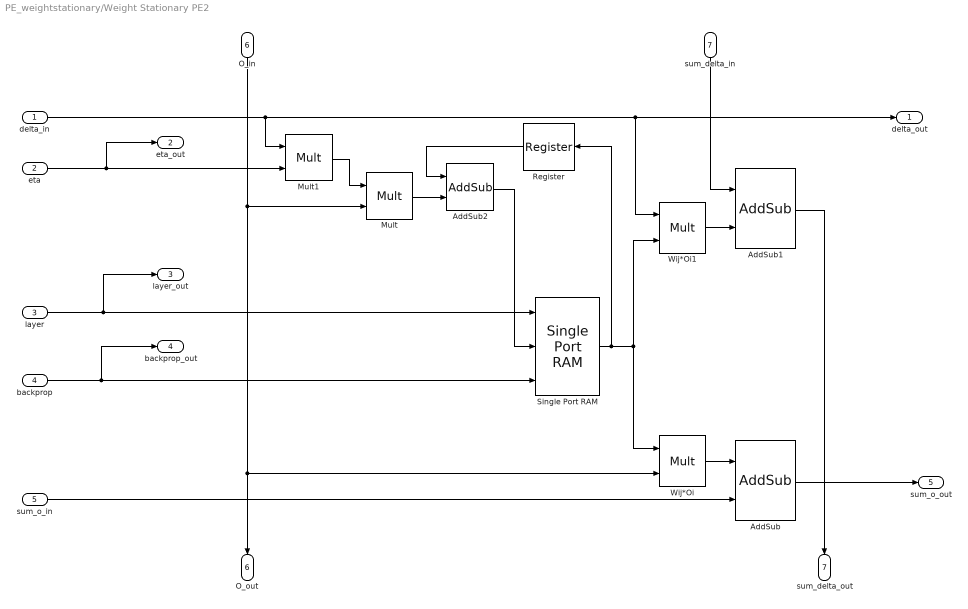
== system PE_weightstationary/Weight Stationary PE2 ==
  delta_in : Inport
  eta : Inport  Port=2
  layer : Inport  Port=3
  backprop : Inport  Port=4
  sum_o_in : Inport  Port=5
  O_in : Inport  Port=6
  sum_delta_in : Inport  Port=7
  AddSub : hdlBasic/AddSub  mode=Addition  use_carryin=off  use_carryout=off  en=off  latency=0  precision=User Defined  arith_type="Signed  (2's comp)"  n_bits=num_bits  bin_pt=frac_bits  quantization=Truncate  overflow=Saturate  use_behavioral_HDL=off  hw_selection=Fabric  pipelined=off  XmcBlockStatus=1  maskContainerNames=tabcontainer1  block_type=addsub  block_config=sysgen:Addsub_config
  AddSub1 : hdlBasic/AddSub  mode=Addition  use_carryin=off  use_carryout=off  en=off  latency=0  precision=User Defined  arith_type="Signed  (2's comp)"  n_bits=num_bits  bin_pt=frac_bits  quantization=Truncate  overflow=Saturate  use_behavioral_HDL=off  hw_selection=Fabric  pipelined=off  XmcBlockStatus=1  maskContainerNames=tabcontainer1  block_type=addsub  block_config=sysgen:Addsub_config
  AddSub2 : hdlBasic/AddSub  mode=Subtraction  use_carryin=off  use_carryout=off  en=off  latency=0  precision=User Defined  arith_type="Signed  (2's comp)"  n_bits=num_bits  bin_pt=frac_bits  quantization=Truncate  overflow=Wrap  use_behavioral_HDL=off  hw_selection=Fabric  pipelined=off  XmcBlockStatus=1  maskContainerNames=tabcontainer1  block_type=addsub  block_config=sysgen:Addsub_config
  Mult : hdlBasic/Mult  precision=User Defined  arith_type="Signed  (2's comp)"  n_bits=num_bits  bin_pt=frac_bits  quantization=Truncate  overflow=Saturate  en=off  latency=0  use_behavioral_HDL=off  opt=Speed  use_embedded=on  optimum_pipeline=off  pipeline=on  use_rpm=on  placement_style=Triangular  XmcBlockStatus=1  maskContainerNames=group1  block_type=mult  block_config=sysgen:Mult_config  block_width=598  block_height=876
  Mult1 : hdlBasic/Mult  precision=User Defined  arith_type="Signed  (2's comp)"  n_bits=num_bits  bin_pt=frac_bits  quantization=Truncate  overflow=Saturate  en=off  latency=0  use_behavioral_HDL=off  opt=Speed  use_embedded=on  optimum_pipeline=off  pipeline=on  use_rpm=on  placement_style=Triangular  XmcBlockStatus=1  maskContainerNames=group1  block_type=mult  block_config=sysgen:Mult_config  block_width=598  block_height=876
  Register : hdlBasic/Register  init=0  rst=off  en=off  XmcBlockStatus=1  maskContainerNames=tabcontainer1  block_type=register  block_config=sysgen:Register_config
  Single Port RAM : hdlBasic/Single Port RAM  depth=num_layer  initVector=initial_weight  distributed_mem=Block RAM  write_mode=Read After Write  rst=off  init_reg=0  en=off  optimize_latency=off  latency=1  optimize=Area  dbl_ovrd=off  simulation_type=fast_sim  XmcBlockStatus=1  maskContainerNames=tabcontainer1  block_type=spram  block_config=sysgen:SPRAM_config
  Wij*Oi : hdlBasic/Mult  precision=User Defined  arith_type="Signed  (2's comp)"  n_bits=num_bits  bin_pt=frac_bits  quantization=Truncate  overflow=Saturate  en=off  latency=0  use_behavioral_HDL=off  opt=Speed  use_embedded=on  optimum_pipeline=off  pipeline=on  use_rpm=on  placement_style=Triangular  XmcBlockStatus=1  maskContainerNames=group1  block_type=mult  block_config=sysgen:Mult_config  block_width=598  block_height=876
  Wij*Oi1 : hdlBasic/Mult  precision=User Defined  arith_type="Signed  (2's comp)"  n_bits=num_bits  bin_pt=frac_bits  quantization=Truncate  overflow=Saturate  en=off  latency=0  use_behavioral_HDL=off  opt=Speed  use_embedded=on  optimum_pipeline=off  pipeline=on  use_rpm=on  placement_style=Triangular  XmcBlockStatus=1  maskContainerNames=group1  block_type=mult  block_config=sysgen:Mult_config  block_width=598  block_height=876
  delta_out : Outport
  eta_out : Outport  Port=2
  layer_out : Outport  Port=3
  backprop_out : Outport  Port=4
  sum_o_out : Outport  Port=5
  O_out : Outport  Port=6
  sum_delta_out : Outport  Port=7
  wires:
  Wij*Oi1/1 -> AddSub1/2
  O_in/1 -> Wij*Oi/2, O_out/1, Mult/2
  Single Port RAM/1 -> Wij*Oi1/2, Wij*Oi/1, Register/1
  Wij*Oi/1 -> AddSub/1
  Mult/1 -> AddSub2/2
  AddSub1/1 -> sum_delta_out/1
  AddSub2/1 -> Single Port RAM/2
  Mult1/1 -> Mult/1
  delta_in/1 -> delta_out/1, Wij*Oi1/1, Mult1/1
  sum_o_in/1 -> AddSub/2
  AddSub/1 -> sum_o_out/1
  eta/1 -> Mult1/2, eta_out/1
  sum_delta_in/1 -> AddSub1/1
  backprop/1 -> Single Port RAM/3, backprop_out/1
  Register/1 -> AddSub2/1
  layer/1 -> Single Port RAM/1, layer_out/1

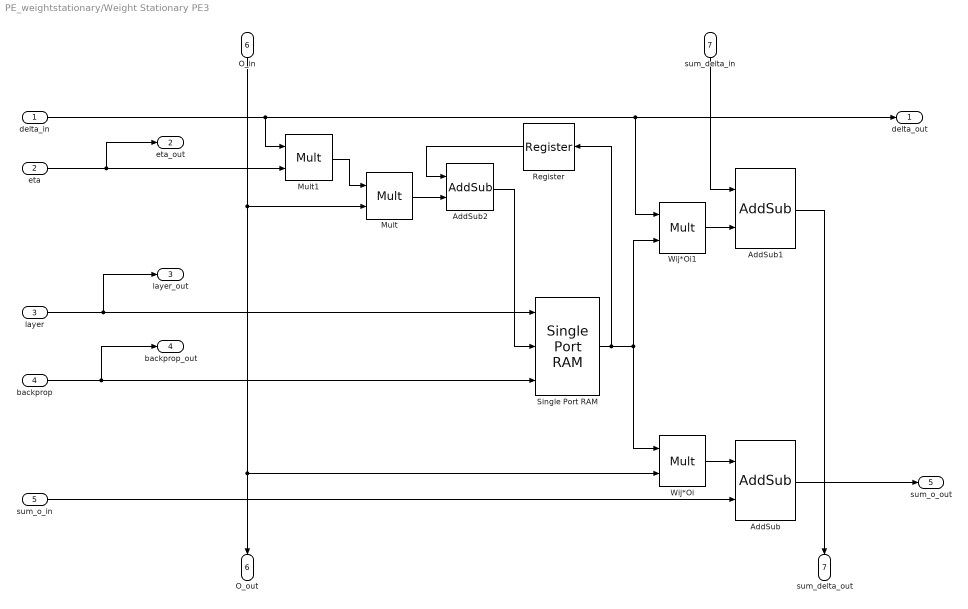
== system PE_weightstationary/Weight Stationary PE3 ==
  delta_in : Inport
  eta : Inport  Port=2
  layer : Inport  Port=3
  backprop : Inport  Port=4
  sum_o_in : Inport  Port=5
  O_in : Inport  Port=6
  sum_delta_in : Inport  Port=7
  AddSub : hdlBasic/AddSub  mode=Addition  use_carryin=off  use_carryout=off  en=off  latency=0  precision=User Defined  arith_type="Signed  (2's comp)"  n_bits=num_bits  bin_pt=frac_bits  quantization=Truncate  overflow=Saturate  use_behavioral_HDL=off  hw_selection=Fabric  pipelined=off  XmcBlockStatus=1  maskContainerNames=tabcontainer1  block_type=addsub  block_config=sysgen:Addsub_config
  AddSub1 : hdlBasic/AddSub  mode=Addition  use_carryin=off  use_carryout=off  en=off  latency=0  precision=User Defined  arith_type="Signed  (2's comp)"  n_bits=num_bits  bin_pt=frac_bits  quantization=Truncate  overflow=Saturate  use_behavioral_HDL=off  hw_selection=Fabric  pipelined=off  XmcBlockStatus=1  maskContainerNames=tabcontainer1  block_type=addsub  block_config=sysgen:Addsub_config
  AddSub2 : hdlBasic/AddSub  mode=Subtraction  use_carryin=off  use_carryout=off  en=off  latency=0  precision=User Defined  arith_type="Signed  (2's comp)"  n_bits=num_bits  bin_pt=frac_bits  quantization=Truncate  overflow=Wrap  use_behavioral_HDL=off  hw_selection=Fabric  pipelined=off  XmcBlockStatus=1  maskContainerNames=tabcontainer1  block_type=addsub  block_config=sysgen:Addsub_config
  Mult : hdlBasic/Mult  precision=User Defined  arith_type="Signed  (2's comp)"  n_bits=num_bits  bin_pt=frac_bits  quantization=Truncate  overflow=Saturate  en=off  latency=0  use_behavioral_HDL=off  opt=Speed  use_embedded=on  optimum_pipeline=off  pipeline=on  use_rpm=on  placement_style=Triangular  XmcBlockStatus=1  maskContainerNames=group1  block_type=mult  block_config=sysgen:Mult_config  block_width=598  block_height=876
  Mult1 : hdlBasic/Mult  precision=User Defined  arith_type="Signed  (2's comp)"  n_bits=num_bits  bin_pt=frac_bits  quantization=Truncate  overflow=Saturate  en=off  latency=0  use_behavioral_HDL=off  opt=Speed  use_embedded=on  optimum_pipeline=off  pipeline=on  use_rpm=on  placement_style=Triangular  XmcBlockStatus=1  maskContainerNames=group1  block_type=mult  block_config=sysgen:Mult_config  block_width=598  block_height=876
  Register : hdlBasic/Register  init=0  rst=off  en=off  XmcBlockStatus=1  maskContainerNames=tabcontainer1  block_type=register  block_config=sysgen:Register_config
  Single Port RAM : hdlBasic/Single Port RAM  depth=num_layer  initVector=initial_weight  distributed_mem=Block RAM  write_mode=Read After Write  rst=off  init_reg=0  en=off  optimize_latency=off  latency=1  optimize=Area  dbl_ovrd=off  simulation_type=fast_sim  XmcBlockStatus=1  maskContainerNames=tabcontainer1  block_type=spram  block_config=sysgen:SPRAM_config
  Wij*Oi : hdlBasic/Mult  precision=User Defined  arith_type="Signed  (2's comp)"  n_bits=num_bits  bin_pt=frac_bits  quantization=Truncate  overflow=Saturate  en=off  latency=0  use_behavioral_HDL=off  opt=Speed  use_embedded=on  optimum_pipeline=off  pipeline=on  use_rpm=on  placement_style=Triangular  XmcBlockStatus=1  maskContainerNames=group1  block_type=mult  block_config=sysgen:Mult_config  block_width=598  block_height=876
  Wij*Oi1 : hdlBasic/Mult  precision=User Defined  arith_type="Signed  (2's comp)"  n_bits=num_bits  bin_pt=frac_bits  quantization=Truncate  overflow=Saturate  en=off  latency=0  use_behavioral_HDL=off  opt=Speed  use_embedded=on  optimum_pipeline=off  pipeline=on  use_rpm=on  placement_style=Triangular  XmcBlockStatus=1  maskContainerNames=group1  block_type=mult  block_config=sysgen:Mult_config  block_width=598  block_height=876
  delta_out : Outport
  eta_out : Outport  Port=2
  layer_out : Outport  Port=3
  backprop_out : Outport  Port=4
  sum_o_out : Outport  Port=5
  O_out : Outport  Port=6
  sum_delta_out : Outport  Port=7
  wires:
  Wij*Oi1/1 -> AddSub1/2
  O_in/1 -> Wij*Oi/2, O_out/1, Mult/2
  Single Port RAM/1 -> Wij*Oi1/2, Wij*Oi/1, Register/1
  Wij*Oi/1 -> AddSub/1
  Mult/1 -> AddSub2/2
  AddSub1/1 -> sum_delta_out/1
  AddSub2/1 -> Single Port RAM/2
  Mult1/1 -> Mult/1
  delta_in/1 -> delta_out/1, Wij*Oi1/1, Mult1/1
  sum_o_in/1 -> AddSub/2
  AddSub/1 -> sum_o_out/1
  eta/1 -> Mult1/2, eta_out/1
  sum_delta_in/1 -> AddSub1/1
  backprop/1 -> Single Port RAM/3, backprop_out/1
  Register/1 -> AddSub2/1
  layer/1 -> Single Port RAM/1, layer_out/1

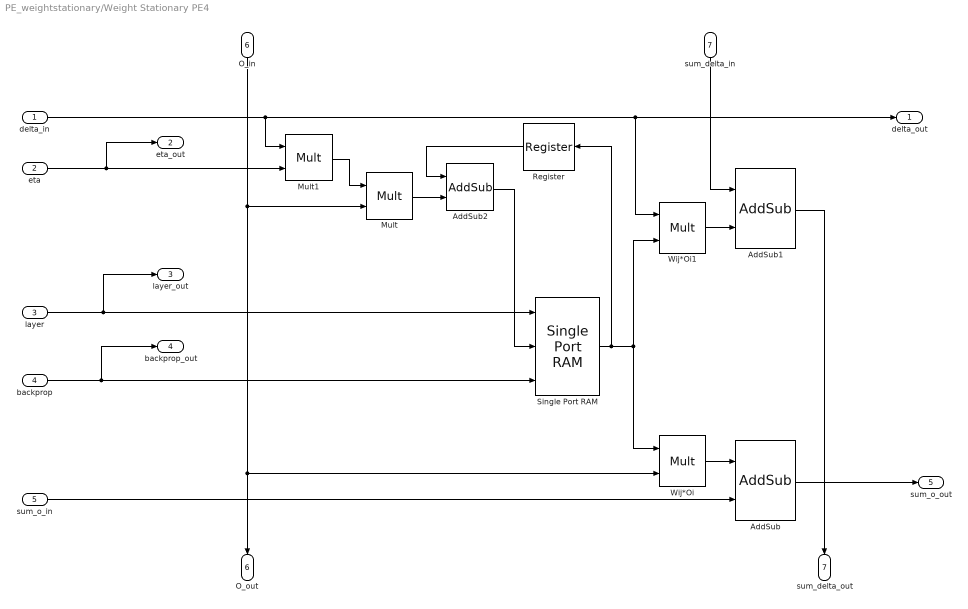
== system PE_weightstationary/Weight Stationary PE4 ==
  delta_in : Inport
  eta : Inport  Port=2
  layer : Inport  Port=3
  backprop : Inport  Port=4
  sum_o_in : Inport  Port=5
  O_in : Inport  Port=6
  sum_delta_in : Inport  Port=7
  AddSub : hdlBasic/AddSub  mode=Addition  use_carryin=off  use_carryout=off  en=off  latency=0  precision=User Defined  arith_type="Signed  (2's comp)"  n_bits=num_bits  bin_pt=frac_bits  quantization=Truncate  overflow=Saturate  use_behavioral_HDL=off  hw_selection=Fabric  pipelined=off  XmcBlockStatus=1  maskContainerNames=tabcontainer1  block_type=addsub  block_config=sysgen:Addsub_config
  AddSub1 : hdlBasic/AddSub  mode=Addition  use_carryin=off  use_carryout=off  en=off  latency=0  precision=User Defined  arith_type="Signed  (2's comp)"  n_bits=num_bits  bin_pt=frac_bits  quantization=Truncate  overflow=Saturate  use_behavioral_HDL=off  hw_selection=Fabric  pipelined=off  XmcBlockStatus=1  maskContainerNames=tabcontainer1  block_type=addsub  block_config=sysgen:Addsub_config
  AddSub2 : hdlBasic/AddSub  mode=Subtraction  use_carryin=off  use_carryout=off  en=off  latency=0  precision=User Defined  arith_type="Signed  (2's comp)"  n_bits=num_bits  bin_pt=frac_bits  quantization=Truncate  overflow=Wrap  use_behavioral_HDL=off  hw_selection=Fabric  pipelined=off  XmcBlockStatus=1  maskContainerNames=tabcontainer1  block_type=addsub  block_config=sysgen:Addsub_config
  Mult : hdlBasic/Mult  precision=User Defined  arith_type="Signed  (2's comp)"  n_bits=num_bits  bin_pt=frac_bits  quantization=Truncate  overflow=Saturate  en=off  latency=0  use_behavioral_HDL=off  opt=Speed  use_embedded=on  optimum_pipeline=off  pipeline=on  use_rpm=on  placement_style=Triangular  XmcBlockStatus=1  maskContainerNames=group1  block_type=mult  block_config=sysgen:Mult_config  block_width=598  block_height=876
  Mult1 : hdlBasic/Mult  precision=User Defined  arith_type="Signed  (2's comp)"  n_bits=num_bits  bin_pt=frac_bits  quantization=Truncate  overflow=Saturate  en=off  latency=0  use_behavioral_HDL=off  opt=Speed  use_embedded=on  optimum_pipeline=off  pipeline=on  use_rpm=on  placement_style=Triangular  XmcBlockStatus=1  maskContainerNames=group1  block_type=mult  block_config=sysgen:Mult_config  block_width=598  block_height=876
  Register : hdlBasic/Register  init=0  rst=off  en=off  XmcBlockStatus=1  maskContainerNames=tabcontainer1  block_type=register  block_config=sysgen:Register_config
  Single Port RAM : hdlBasic/Single Port RAM  depth=num_layer  initVector=initial_weight  distributed_mem=Block RAM  write_mode=Read Before Write  rst=off  init_reg=0  en=off  optimize_latency=off  latency=1  optimize=Area  dbl_ovrd=off  simulation_type=fast_sim  XmcBlockStatus=1  maskContainerNames=tabcontainer1  block_type=spram  block_config=sysgen:SPRAM_config
  Wij*Oi : hdlBasic/Mult  precision=User Defined  arith_type="Signed  (2's comp)"  n_bits=num_bits  bin_pt=frac_bits  quantization=Truncate  overflow=Saturate  en=off  latency=0  use_behavioral_HDL=off  opt=Speed  use_embedded=on  optimum_pipeline=off  pipeline=on  use_rpm=on  placement_style=Triangular  XmcBlockStatus=1  maskContainerNames=group1  block_type=mult  block_config=sysgen:Mult_config  block_width=598  block_height=876
  Wij*Oi1 : hdlBasic/Mult  precision=User Defined  arith_type="Signed  (2's comp)"  n_bits=num_bits  bin_pt=frac_bits  quantization=Truncate  overflow=Saturate  en=off  latency=0  use_behavioral_HDL=off  opt=Speed  use_embedded=on  optimum_pipeline=off  pipeline=on  use_rpm=on  placement_style=Triangular  XmcBlockStatus=1  maskContainerNames=group1  block_type=mult  block_config=sysgen:Mult_config  block_width=598  block_height=876
  delta_out : Outport
  eta_out : Outport  Port=2
  layer_out : Outport  Port=3
  backprop_out : Outport  Port=4
  sum_o_out : Outport  Port=5
  O_out : Outport  Port=6
  sum_delta_out : Outport  Port=7
  wires:
  Wij*Oi1/1 -> AddSub1/2
  O_in/1 -> Wij*Oi/2, O_out/1, Mult/2
  Single Port RAM/1 -> Wij*Oi1/2, Wij*Oi/1, Register/1
  Wij*Oi/1 -> AddSub/1
  Mult/1 -> AddSub2/2
  AddSub1/1 -> sum_delta_out/1
  AddSub2/1 -> Single Port RAM/2
  Mult1/1 -> Mult/1
  delta_in/1 -> delta_out/1, Wij*Oi1/1, Mult1/1
  sum_o_in/1 -> AddSub/2
  AddSub/1 -> sum_o_out/1
  eta/1 -> Mult1/2, eta_out/1
  sum_delta_in/1 -> AddSub1/1
  backprop/1 -> Single Port RAM/3, backprop_out/1
  Register/1 -> AddSub2/1
  layer/1 -> Single Port RAM/1, layer_out/1
